simulink model "airspeed_pitch"  (R2017a)
settings: Solver=VariableStepAuto  StartTime=0.0  StopTime=100  RelTol=1e-3
undefined symbols (not defined in the file): a_V1, P
settings Model: Creator=pizzaslayer  LastModifiedBy=Parth

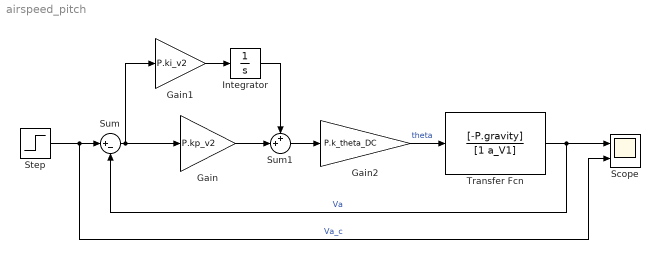
== system airspeed_pitch ==
  Gain : Gain  Gain=P.kp_v2
  Gain1 : Gain  Gain=P.ki_v2
  Gain2 : Gain  Gain=P.k_theta_DC
  Integrator : Integrator
  Scope : Scope  NumInputPorts=2
  Step : Step  Time=0  Before=.1  After=.8  SampleTime=0
  Sum : Sum  Inputs=|+-
  Sum1 : Sum  Inputs=++|
  Transfer Fcn : TransferFcn  Numerator=[-P.gravity]  Denominator=[1 a_V1]
  wires:
  Step/1 -> Scope/2, Sum/1  "Va_c"
  Gain1/1 -> Integrator/1
  Sum/1 -> Gain/1, Gain1/1
  Integrator/1 -> Sum1/1
  Gain/1 -> Sum1/2
  Sum1/1 -> Gain2/1
  Gain2/1 -> Transfer Fcn/1  "theta"
  Transfer Fcn/1 -> Sum/2, Scope/1  "Va"
